simulink model "robotController"  (R2020b)
settings: Solver=FixedStepAuto  StartTime=0.0  StopTime=10.0  FixedStep=0.1  RelTol=1e-3
PostLoadFcn:
  | set_param(gcs, 'ForceConsistencyChecking', 'off');
InitFcn:
  | set_param('robotController', 'ForceConsistencyChecking', 'off');
values from neighbouring files (symbols this model uses):
  awayFromGoalThresh = 0.7    [example.m]    (also in warehouseInitial.mat)
  logicalMap = [1 1 1 1 1 1 1 1 1 1 1 1 ... (10000 elements, 100x100)]    [warehouseInitial.mat]
libraries: robotalgslib x2
settings Model: OrderedModelArguments=off  Creator=The MathWorks, Inc.  LastModifiedBy=fan

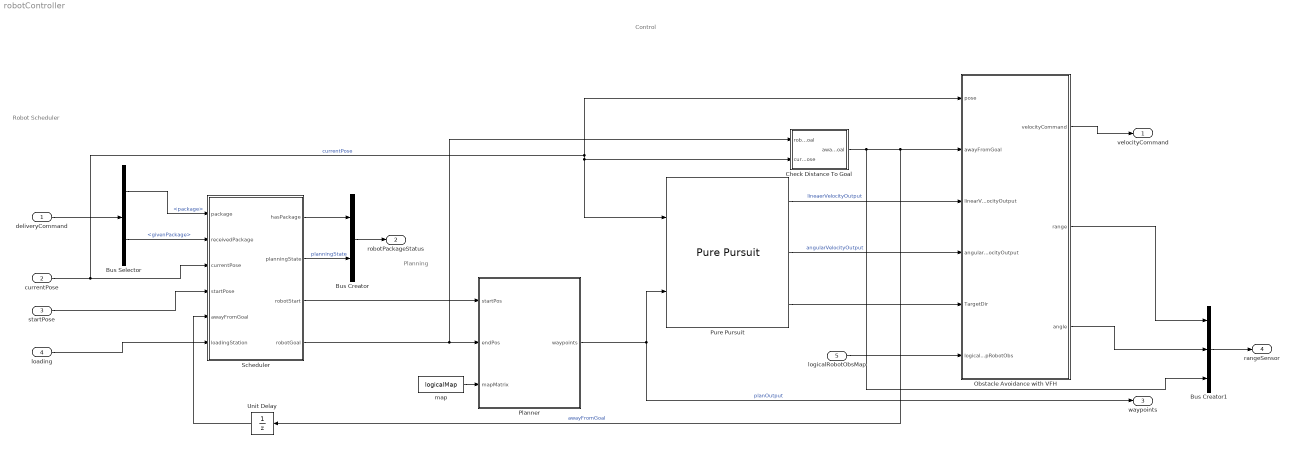
== system robotController ==
  note: Control
  note: Planning
  note: Robot Scheduler
  deliveryCommand : Inport  OutDataTypeStr=Bus: RobotDeliverCommand  BusOutputAsStruct=on
  currentPose : Inport  Port=2  PortDimensions=[3, 1]
  startPose : Inport  Port=3
  loading : Inport  Port=4
  logicalRobotObsMap : Inport  Port=5  OutDataTypeStr=boolean  PortDimensions=[100,100]
  Bus Creator : BusCreator  Inputs=2  OutDataTypeStr=Bus: RobotPackageStatus  NonVirtualBus=on
      settings: InheritFromInputs=off
  Bus Creator1 : BusCreator  Inputs=3  OutDataTypeStr=Bus: RangeSensor  NonVirtualBus=on
  Bus Selector : BusSelector  OutputSignals=package,givenPackage
  Check Distance To Goal : Subsystem
  Obstacle Avoidance with VFH : Subsystem
  Planner : MATLAB Function  TreatAsAtomicUnit=on
  Pure Pursuit : robotalgslib/Pure Pursuit  DesiredLinearVelocity=0.1  MaxAngularVelocity=1.0  LookaheadDistance=1.2  TargetDirPort=on  SimulateUsing=Code generation
  Scheduler : Stateflow chart  Priority=2
  Unit Delay : UnitDelay  SampleTime=-1  HasFrameUpgradeWarning=on
  map : Constant  Value=logicalMap
  velocityCommand : Outport
  robotPackageStatus : Outport  Port=2  OutDataTypeStr=Bus: RobotPackageStatus  BusOutputAsStruct=on
  waypoints : Outport  Port=3
  rangeSensor : Outport  Port=4  OutDataTypeStr=Bus: RangeSensor  BusOutputAsStruct=on
  wires:
  Scheduler/2(planningState) -> Bus Creator/2  "planningState"
  Check Distance To Goal/1(awayFromGoal) -> Unit Delay/1, Obstacle Avoidance with VFH/2(awayFromGoal), Bus Creator1/3  "awayFromGoal"
  Bus Selector/2 -> Scheduler/2(receivedPackage)  "<givenPackage>"
  Obstacle Avoidance with VFH/1(velocityCommand) -> velocityCommand/1
  currentPose/1 -> Pure Pursuit/1, Check Distance To Goal/2(currentPose), Obstacle Avoidance with VFH/1(pose), Scheduler/3(currentPose)  "currentPose"
  Unit Delay/1 -> Scheduler/5(awayFromGoal)
  Scheduler/1(hasPackage) -> Bus Creator/1
  Planner/1(waypoints) -> Pure Pursuit/2, waypoints/1  "planOutput"
  startPose/1 -> Scheduler/4(startPose)
  Bus Creator/1 -> robotPackageStatus/1
  map/1 -> Planner/3(mapMatrix)
  Scheduler/4(robotGoal) -> Planner/2(endPos), Check Distance To Goal/1(robotGoal)
  Bus Selector/1 -> Scheduler/1(package)  "<package>"
  deliveryCommand/1 -> Bus Selector/1
  Scheduler/3(robotStart) -> Planner/1(startPos)
  loading/1 -> Scheduler/6(loadingStation)
  Pure Pursuit/3 -> Obstacle Avoidance with VFH/5(TargetDir)
  Pure Pursuit/2 -> Obstacle Avoidance with VFH/4(angularVelocityOutput)  "angularVelocityOutput"
  Pure Pursuit/1 -> Obstacle Avoidance with VFH/3(linearVelocityOutput)  "lineaerVelocityOutput"
  logicalRobotObsMap/1 -> Obstacle Avoidance with VFH/6(logicalMapRobotObs)
  Obstacle Avoidance with VFH/2(range) -> Bus Creator1/1
  Obstacle Avoidance with VFH/3(angle) -> Bus Creator1/2
  Bus Creator1/1 -> rangeSensor/1

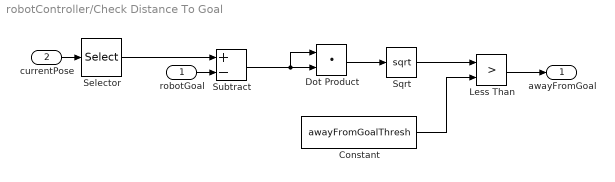
== system robotController/Check Distance To Goal ==
  robotGoal : Inport
  currentPose : Inport  Port=2
  Constant : Constant  Value=awayFromGoalThresh
  Dot Product : DotProduct  InputSameDT=on  OutDataTypeStr=Inherit: Inherit via internal rule
  Less Than : RelationalOperator  Operator=>  OutDataTypeStr=boolean  RndMeth=Simplest
  Selector : Selector  InputPortWidth=3  IndexOptions=Index vector (dialog)  Indices=[1 2]  OutputSizes=1
  Sqrt : Sqrt  SaturateOnIntegerOverflow=on
  Subtract : Sum  Inputs=+-
  awayFromGoal : Outport  OutDataTypeStr=boolean
  wires:
  robotGoal/1 -> Subtract/2
  Dot Product/1 -> Sqrt/1
  Constant/1 -> Less Than/2
  currentPose/1 -> Selector/1
  Less Than/1 -> awayFromGoal/1
  Sqrt/1 -> Less Than/1
  Subtract/1 -> Dot Product/1, Dot Product/2
  Selector/1 -> Subtract/1

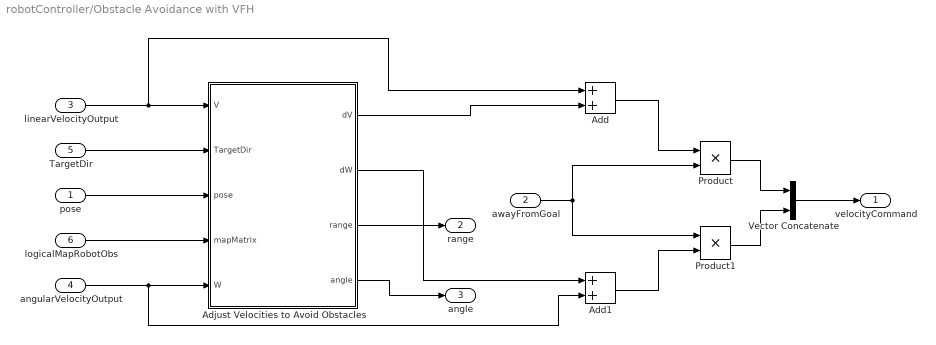
== system robotController/Obstacle Avoidance with VFH ==
  pose : Inport
  awayFromGoal : Inport  Port=2  OutDataTypeStr=boolean
  linearVelocityOutput : Inport  Port=3
  angularVelocityOutput : Inport  Port=4
  TargetDir : Inport  Port=5
  logicalMapRobotObs : Inport  Port=6
  Add : Sum
  Add1 : Sum
  Adjust Velocities to Avoid Obstacles : Subsystem
  Product : Product
  Product1 : Product
  Vector Concatenate : Concatenate
  velocityCommand : Outport  OutDataTypeStr=double
  range : Outport  Port=2
  angle : Outport  Port=3
  wires:
  awayFromGoal/1 -> Product/2, Product1/1
  Adjust Velocities to Avoid Obstacles/2(dW) -> Add1/1
  angularVelocityOutput/1 -> Adjust Velocities to Avoid Obstacles/5(W), Add1/2
  Add1/1 -> Product1/2
  Add/1 -> Product/1
  logicalMapRobotObs/1 -> Adjust Velocities to Avoid Obstacles/4(mapMatrix)
  linearVelocityOutput/1 -> Add/1, Adjust Velocities to Avoid Obstacles/1(V)
  Adjust Velocities to Avoid Obstacles/1(dV) -> Add/2
  TargetDir/1 -> Adjust Velocities to Avoid Obstacles/2(TargetDir)
  pose/1 -> Adjust Velocities to Avoid Obstacles/3(pose)
  Product/1 -> Vector Concatenate/1
  Product1/1 -> Vector Concatenate/2
  Vector Concatenate/1 -> velocityCommand/1
  Adjust Velocities to Avoid Obstacles/3(range) -> range/1
  Adjust Velocities to Avoid Obstacles/4(angle) -> angle/1

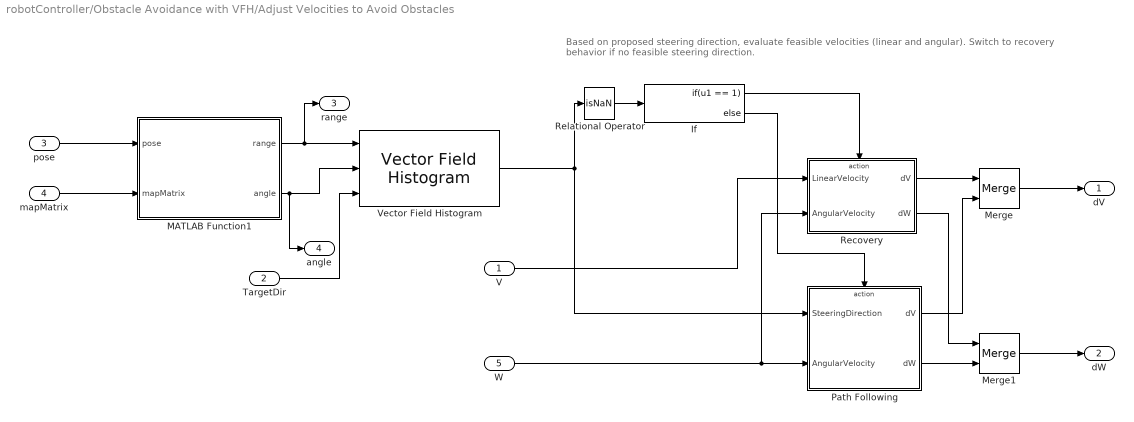
== system robotController/Obstacle Avoidance with VFH/Adjust Velocities to Avoid Obstacles ==
  note: Based on proposed steering direction, evaluate feasible velocities (linear and angular).
      | 				Switch to recovery behavior if no feasible steering direction.
  V : Inport
  TargetDir : Inport  Port=2
  pose : Inport  Port=3
  mapMatrix : Inport  Port=4
  W : Inport  Port=5
  If : If  IfExpression=u1 == 1
  MATLAB Function1 : MATLAB Function  TreatAsAtomicUnit=on
  Merge : Merge
  Merge1 : Merge
  Path Following : Subsystem  TreatAsAtomicUnit=on
  Recovery : Subsystem  TreatAsAtomicUnit=on
  Relational Operator : RelationalOperator  Operator=isNaN  OutDataTypeStr=boolean  RndMeth=Simplest
  Vector Field Histogram : robotalgslib/Vector Field Histogram  NumAngularSectors=180  DistanceLimits=[ 0.05, 3]  HistogramThresholds=[ 3, 8 ]  RobotRadius=0.5  SafetyDistance=1  MinTurningRadius=0.5  SimulateUsing=Code generation  TargetDirectionWeight=5  CurrentDirectionWeight=2  PreviousDirectionWeight=2
      settings: SourceProductBaseCode=NV,RO
  dV : Outport  VectorParamsAs1DForOutWhenUnconnected=off
  dW : Outport  Port=2  VectorParamsAs1DForOutWhenUnconnected=off
  range : Outport  Port=3  VectorParamsAs1DForOutWhenUnconnected=off
  angle : Outport  Port=4  VectorParamsAs1DForOutWhenUnconnected=off
  wires:
  Merge1/1 -> dW/1
  V/1 -> Recovery/1(LinearVelocity)
  W/1 -> Recovery/2(AngularVelocity), Path Following/2(AngularVelocity)
  Relational Operator/1 -> If/1
  Merge/1 -> dV/1
  If/1 -> Recovery/Action
  If/2 -> Path Following/Action
  Recovery/2(dW) -> Merge1/1
  Path Following/2(dW) -> Merge1/2
  Recovery/1(dV) -> Merge/1
  Path Following/1(dV) -> Merge/2
  pose/1 -> MATLAB Function1/1(pose)
  mapMatrix/1 -> MATLAB Function1/2(mapMatrix)
  Vector Field Histogram/1 -> Path Following/1(SteeringDirection), Relational Operator/1
  MATLAB Function1/1(range) -> range/1, Vector Field Histogram/1
  MATLAB Function1/2(angle) -> angle/1, Vector Field Histogram/2
  TargetDir/1 -> Vector Field Histogram/3

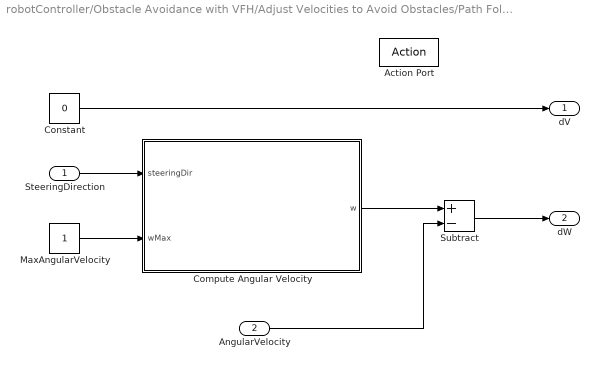
== system robotController/Obstacle Avoidance with VFH/Adjust Velocities to Avoid Obstacles/Path Following ==
  SteeringDirection : Inport
  AngularVelocity : Inport  Port=2
  Action Port : ActionPort  ActionPortLabel=else
  Compute Angular Velocity : MATLAB Function  TreatAsAtomicUnit=on
  Constant : Constant  Value=0
  MaxAngularVelocity : Constant
  Subtract : Sum  Inputs=+-
  dV : Outport  VectorParamsAs1DForOutWhenUnconnected=off
  dW : Outport  Port=2  VectorParamsAs1DForOutWhenUnconnected=off
  wires:
  Constant/1 -> dV/1
  MaxAngularVelocity/1 -> Compute Angular Velocity/2(wMax)
  SteeringDirection/1 -> Compute Angular Velocity/1(steeringDir)
  Subtract/1 -> dW/1
  Compute Angular Velocity/1(w) -> Subtract/1
  AngularVelocity/1 -> Subtract/2

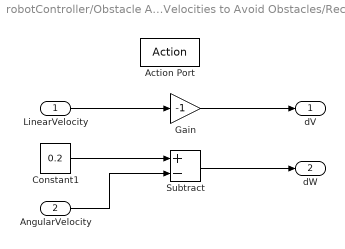
== system robotController/Obstacle Avoidance with VFH/Adjust Velocities to Avoid Obstacles/Recovery ==
  LinearVelocity : Inport
  AngularVelocity : Inport  Port=2
  Action Port : ActionPort  ActionPortLabel=if(u1 == 1)
  Constant1 : Constant  Value=0.2
  Gain : Gain  Gain=-1
  Subtract : Sum  Inputs=+-
  dV : Outport  VectorParamsAs1DForOutWhenUnconnected=off
  dW : Outport  Port=2  VectorParamsAs1DForOutWhenUnconnected=off
  wires:
  LinearVelocity/1 -> Gain/1
  Gain/1 -> dV/1
  Constant1/1 -> Subtract/1
  AngularVelocity/1 -> Subtract/2
  Subtract/1 -> dW/1

== matlab function robotController/Planner ==
  settings: updateMethod=DISCRETE
  data: startPos input size=[1 2]; endPos input size=[1 2]; waypoints output size=[100 2]; mapMatrix input
function waypoints = planning(startPos, endPos, mapMatrix)

persistent waypointsInternal
persistent prevStartPos
persistent prevEndPos

% Set constant parameters
maxNumNodes = 100;

% Initialize persistent variables that are used downstream
if isempty(prevStartPos)
    prevStartPos = startPos;
end

if isempty(prevEndPos)
    prevEndPos = endPos;
end

isNewPath = (~isequal(prevStartPos, startPos) || ~isequal(prevEndPos, endPos));

if isempty(waypointsInternal) || isNewPath
    % Two conditions in which waypoints must be set: they are not yet
    % initialized, or they are initialized, but the current start and end
    % do not match those used to generate the previous set of waypoints
    [waypointsInternal] = planPath(mapMatrix, maxNumNodes, startPos, endPos);
end

% Update the outputs
waypoints = waypointsInternal;

% Update the persistent variables that indicate previous state
prevStartPos = startPos;
prevEndPos = endPos;

%% Helper Function



end

function wayPoints = planPath(mapMatrix, maxNodes, startPos, endPos)
    
    % Create a probabilistic roadmap
    map = binaryOccupancyMap(mapMatrix);
%     prm = mobileRobotPRM(map, maxNodes);
    prm = mobileRobotPRM(map);
    prm.NumNodes = 500;
    
    % Find a path between two points
    xy = findpath(prm, startPos, endPos);
    wayPoints = repmat(endPos, maxNodes, 1);
    
    % Number of nodes that are actually used
    numNodes = length(xy);
    if numNodes <=2 
        disp('no path');
    end
    wayPoints(1:numNodes,:) = xy;    

end

== stateflow chart robotController/Scheduler ==
  settings: sampleTime=0.1
  state GoToUnloadingStation
    entry:
    robotGoal = unloadingStations(package, :)';
    robotStart = currentPose(1:2)';
  state GoToLoadingStation
    entry:
    robotGoal = loadingStation';
    robotStart = currentPose(1:2)';
  state StationHalt
    entry, during:
  state GoToChargingStation
    entry:
    robotGoal = startPose';
    robotStart = currentPose(1:2)';
  (default) -> (junction 65) : {robotStart = startPose;
      | hasPackage = 0;
      | }
  (junction 65) -> GoToLoadingStation
  GoToLoadingStation -> StationHalt [order 1] : [hasPackage && package]
  StationHalt -> GoToUnloadingStation [order 1] : [planningState == RobotState.AtLoadingStn && ...
      | after(stopDelay, tick)]
  GoToUnloadingStation -> StationHalt : [~awayFromGoal]
      | {planningState = RobotState.AtUnloadingStn;
      | hasPackage = 0;}
  GoToLoadingStation -> (junction 72) [order 2] : [~awayFromGoal]{planningState = RobotState.AtLoadingStn;}
  StationHalt -> GoToChargingStation [order 2] : [planningState == RobotState.AtUnloadingStn && ...
      | after(stopDelay, tick)]
  GoToChargingStation -> (junction 116) : [~awayFromGoal]{planningState = RobotState.AtDock;}
  (junction 72) -> (junction 102) : [receivedPackage]{hasPackage = 1;}
  data: hasPackage output; planningState output Enum: RobotState =RobotState.AtDock; robotStart output size=[1, 2]; robotGoal output size=2; unloadingStations parameter; package input; receivedPackage input; currentPose input; startPose input size=[1 2]; awayFromGoal input; stopDelay local =0.5e3; loadingStation input size=[1 2]

== matlab function robotController/Obstacle Avoidance with VFH/Adjust Velocities to Avoid Obstacles/MATLAB Function1 ==
  settings: updateMethod=DISCRETE
  data: range output; pose input size=[3, 1]; mapMatrix input; angle output
function [range, angle]  = RangeSensor(pose, mapMatrix)
persistent r
if isempty(r)
 r = rangeSensor('HorizontalAngle', [-pi/2, pi/2], 'HorizontalAngleResolution', pi/20, 'Range', [0 12]);
end
% remove the obstacle defined in robot's pose
obs_grid = world2grid(binaryOccupancyMap(mapMatrix), pose(1:2)');
mapMatrix(obs_grid(1), obs_grid(2)) = false;
[range, angle] = r(pose', binaryOccupancyMap(mapMatrix, 1));


end

== matlab function robotController/Obstacle Avoidance with VFH/Adjust Velocities to Avoid Obstacles/Path Following/Compute Angular Velocity ==
  data: steeringDir input; w output; wMax input
function w = ComputeAngularVelocity(steeringDir, wMax)

% Allow variable input arguments
if nargin == 1   
    wMax = inf;
end

validateattributes(steeringDir, {'double'},{'real'},...
    'exampleHelperComputeAngularVelocity', 'STEERINGDIR', 1);
validateattributes(wMax, {'double'},{'real', 'positive'},...
    'exampleHelperComputeAngularVelocity', 'WMAX', 2);

% Computing in robot's coordinate frame
curPose = [0 0 0];

% The following computation is similar to robotics.PurePursuit
lookaheadPoint = [cos(steeringDir), sin(steeringDir)];
slope = atan2((lookaheadPoint(2) - curPose(2)), ...
    (lookaheadPoint(1) - curPose(1)));
alpha = angdiff(curPose(3), slope);

% Angular velocity command for a differential drive robot is
% equal to the desired curvature to be followed by the robot.

w = (2*sin(alpha));

% Pick a constant rotation when robot is facing in the opposite
% direction of the path
if abs(abs(alpha) - pi) < 1e-12
    w = sign(w)*1;
end

if abs(w) > wMax
    w = sign(w)*wMax;
end

end
